simulink model "parallel_decimation_testbench_8inputs"  (Simulink 7.4)
settings: Solver=ode45  StartTime=0.0  StopTime=100  RelTol=1e-3
libraries: xbsIndex_r4 x49, simulink x2
settings Model: Creator=chenhong  LastModifiedBy=chenhong

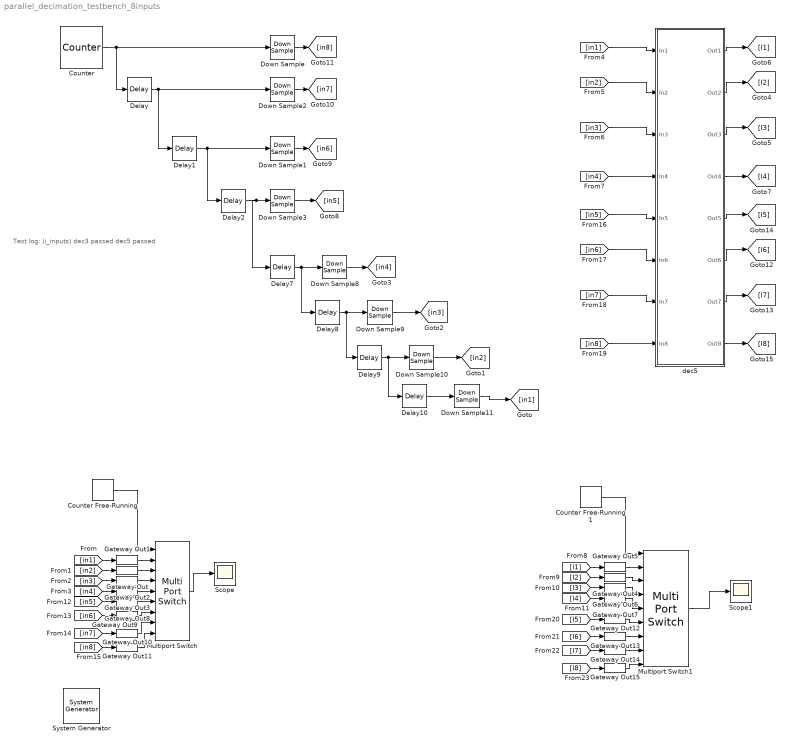
== system parallel_decimation_testbench_8inputs ==
  note: Test log: (i_inputs)
      | dec3 passed
      | dec5 passed
  " System Generator" : xbsIndex_r4/ System Generator  Tag=genX  SystemSampleTime=-1  xilinxfamily=Virtex6  part=xc6vsx315t  speed=-3  package=ff1156  synthesis_tool=XST  clock_wrapper=Clock Enables  directory=./netlist  testbench=off  simulink_period=1  sysclk_period=10  dcm_input_clock_period=10  incr_netlist=off  trim_vbits=Everywhere in SubSystem  dbl_ovrd=According to Block Masks  core_generation=According to Block Masks  run_coregen=off  deprecated_control=off  eval_field=0  block_type=sysgen
      settings: block_version=11.4
  Counter : xbsIndex_r4/Counter  cnt_type=Free Running  cnt_to=Inf  operation=Up  start_count=0  cnt_by_val=1  arith_type=Unsigned  n_bits=8  bin_pt=0  load_pin=off  rst=off  en=off  explicit_period=on  period=1  dbl_ovrd=off  use_behavioral_HDL=off  implementation=Fabric  block_type=counter
      settings: block_version=11.4
  Counter Free-Running : simulink/Sources/Counter Free-Running  SystemSampleTime=-1  NumBits=3  tsamp=1
  Counter Free-Running1 : simulink/Sources/Counter Free-Running  SystemSampleTime=-1  NumBits=3  tsamp=5
  Delay{,1..2,7..10} (7 alike) : xbsIndex_r4/Delay  en=off  latency=1  dbl_ovrd=off  reg_retiming=off  block_type=delay
      settings: block_version=11.4
  Down Sample{,1..3,8..11} (8 alike) : xbsIndex_r4/Down Sample  sample_ratio=8  sample_phase="Last Value of Frame  (most efficient)"  en=off  latency=1  dbl_ovrd=off  block_type=dsamp
      settings: block_version=11.4
  Gateway Out{,1..15} (16 alike) : xbsIndex_r4/Gateway Out  hdl_port=off  timing_constraint=None  locs_specified=off  LOCs={}  block_type=gatewayout
      settings: infoedit="Gateway out block.  Converts Xilinx fixed point inputs into ouputs of type Simulink integer, double, or fixed point.<br><br>Hardware notes:  In hardware these blocks become top level output ports or are discarded, depending on how they are configured."  block_version=11.4
  Multiport Switch : MultiPortSwitch  Inputs=8  zeroidx=on  OutDataType=fixdt(1, 16)  OutScaling=2^0  SampleTime=1
  Multiport Switch1 : MultiPortSwitch  Inputs=8  zeroidx=on  OutDataType=fixdt(1, 16)  OutScaling=2^0  SampleTime=5
  Scope : Scope
  Scope1 : Scope
  dec5 : Subsystem
  wires:
  Counter/1 -> Down Sample/1, Delay/1
  Delay/1 -> Down Sample2/1, Delay1/1
  Delay1/1 -> Down Sample1/1, Delay2/1
  Delay2/1 -> Down Sample3/1, Delay7/1
  Counter Free-Running/1 -> Multiport Switch/1
  Down Sample/1 -> [in8]
  Down Sample2/1 -> [in7]
  Down Sample1/1 -> [in6]
  Down Sample3/1 -> [in5]
  [in1] -> Gateway Out1/1
  [in2] -> Gateway Out/1
  [in3] -> Gateway Out2/1
  [in4] -> Gateway Out3/1
  Gateway Out1/1 -> Multiport Switch/2
  Gateway Out/1 -> Multiport Switch/3
  Gateway Out2/1 -> Multiport Switch/4
  Gateway Out3/1 -> Multiport Switch/5
  Multiport Switch/1 -> Scope/1
  [in2] -> dec5/2(In2)
  [in3] -> dec5/3(In3)
  [in1] -> dec5/1(In1)
  [in4] -> dec5/4(In4)
  dec5/2(Out2) -> [I2]
  dec5/3(Out3) -> [I3]
  dec5/1(Out1) -> [I1]
  dec5/4(Out4) -> [I4]
  Counter Free-Running1/1 -> Multiport Switch1/1
  [I1] -> Gateway Out5/1
  [I2] -> Gateway Out4/1
  [I3] -> Gateway Out6/1
  [I4] -> Gateway Out7/1
  Gateway Out5/1 -> Multiport Switch1/2
  Gateway Out4/1 -> Multiport Switch1/3
  Gateway Out6/1 -> Multiport Switch1/4
  Gateway Out7/1 -> Multiport Switch1/5
  Multiport Switch1/1 -> Scope1/1
  Delay7/1 -> Down Sample8/1, Delay8/1
  Delay8/1 -> Down Sample9/1, Delay9/1
  Delay9/1 -> Down Sample10/1, Delay10/1
  Delay10/1 -> Down Sample11/1
  Down Sample11/1 -> [in1]
  Down Sample10/1 -> [in2]
  Down Sample9/1 -> [in3]
  Down Sample8/1 -> [in4]
  [in5] -> Gateway Out8/1
  Gateway Out8/1 -> Multiport Switch/6
  [in6] -> Gateway Out9/1
  [in7] -> Gateway Out10/1
  [in8] -> Gateway Out11/1
  Gateway Out9/1 -> Multiport Switch/7
  Gateway Out10/1 -> Multiport Switch/8
  Gateway Out11/1 -> Multiport Switch/9
  [in6] -> dec5/6(In6)
  [in7] -> dec5/7(In7)
  [in5] -> dec5/5(In5)
  [in8] -> dec5/8(In8)
  dec5/6(Out6) -> [I6]
  dec5/7(Out7) -> [I7]
  dec5/5(Out5) -> [I5]
  dec5/8(Out8) -> [I8]
  [I5] -> Gateway Out12/1
  [I6] -> Gateway Out13/1
  [I7] -> Gateway Out14/1
  [I8] -> Gateway Out15/1
  Gateway Out12/1 -> Multiport Switch1/6
  Gateway Out13/1 -> Multiport Switch1/7
  Gateway Out14/1 -> Multiport Switch1/8
  Gateway Out15/1 -> Multiport Switch1/9

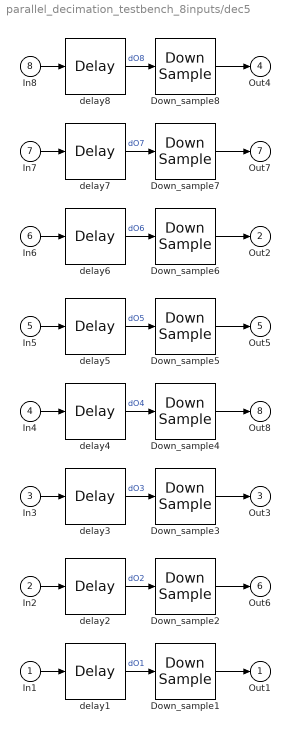
== system parallel_decimation_testbench_8inputs/dec5 ==
  In1 : Inport
  In2 : Inport  Port=2
  In3 : Inport  Port=3
  In4 : Inport  Port=4
  In5 : Inport  Port=5
  In6 : Inport  Port=6
  In7 : Inport  Port=7
  In8 : Inport  Port=8
  Down_sample{1..8} (8 alike) : xbsIndex_r4/Down Sample  sample_ratio=5  sample_phase="Last Value of Frame  (most efficient)"  en=off  latency=1  dbl_ovrd=off  block_type=dsamp
      settings: block_version=11.4
  delay1 : xbsIndex_r4/Delay  en=off  latency=4  dbl_ovrd=off  reg_retiming=off  block_type=delay
      settings: block_version=11.4
  delay2 : xbsIndex_r4/Delay  en=off  latency=1  dbl_ovrd=off  reg_retiming=off  block_type=delay
      settings: block_version=11.4
  delay3 : xbsIndex_r4/Delay  en=off  latency=3  dbl_ovrd=off  reg_retiming=off  block_type=delay
      settings: block_version=11.4
  delay4 : xbsIndex_r4/Delay  en=off  latency=0  dbl_ovrd=off  reg_retiming=off  block_type=delay
      settings: block_version=11.4
  delay5 : xbsIndex_r4/Delay  en=off  latency=2  dbl_ovrd=off  reg_retiming=off  block_type=delay
      settings: block_version=11.4
  delay6 : xbsIndex_r4/Delay  en=off  latency=4  dbl_ovrd=off  reg_retiming=off  block_type=delay
      settings: block_version=11.4
  delay7 : xbsIndex_r4/Delay  en=off  latency=1  dbl_ovrd=off  reg_retiming=off  block_type=delay
      settings: block_version=11.4
  delay8 : xbsIndex_r4/Delay  en=off  latency=3  dbl_ovrd=off  reg_retiming=off  block_type=delay
      settings: block_version=11.4
  Out1 : Outport
  Out2 : Outport  Port=2
  Out3 : Outport  Port=3
  Out4 : Outport  Port=4
  Out5 : Outport  Port=5
  Out6 : Outport  Port=6
  Out7 : Outport  Port=7
  Out8 : Outport  Port=8
  wires:
  delay8/1 -> Down_sample8/1  "dO8"
  In8/1 -> delay8/1
  Down_sample7/1 -> Out7/1
  delay6/1 -> Down_sample6/1  "dO6"
  In6/1 -> delay6/1
  Down_sample5/1 -> Out5/1
  delay4/1 -> Down_sample4/1  "dO4"
  In4/1 -> delay4/1
  Down_sample3/1 -> Out3/1
  delay2/1 -> Down_sample2/1  "dO2"
  In2/1 -> delay2/1
  Down_sample1/1 -> Out1/1
  In1/1 -> delay1/1
  delay1/1 -> Down_sample1/1  "dO1"
  Down_sample2/1 -> Out6/1
  In3/1 -> delay3/1
  delay3/1 -> Down_sample3/1  "dO3"
  Down_sample4/1 -> Out8/1
  In5/1 -> delay5/1
  delay5/1 -> Down_sample5/1  "dO5"
  Down_sample6/1 -> Out2/1
  In7/1 -> delay7/1
  delay7/1 -> Down_sample7/1  "dO7"
  Down_sample8/1 -> Out4/1
